simulink model "system_simulink-1"  (R2021b)
settings: Solver=ode45  StartTime=0.0  StopTime=20  RelTol=1e-3  EnableMultiTasking=on
undefined symbols (not defined in the file): dynamic_pre_comp, K, k_d, static_compensator
settings Model: Creator=Cabral  LastModifiedBy=Mohammad masih
settings SolverCC: AlgebraicLoopSolver=TrustRegion
settings DataIOCC: LimitDataPoints=on  SaveFormat=Array  SignalLoggingSaveFormat=ModelDataLogs  ReturnWorkspaceOutputs=off
settings OptimizationCC: ExpressionDepthLimit=2147483647  InitFltsAndDblsToZero=on  LifeSpan=inf
settings DebuggingCC: SaveWithParameterizedLinksMsg=none  UnderspecifiedInitializationDetection=Classic  MergeDetectMultiDrivingBlocksExec=none  SignalResolutionControl=TryResolveAllWithWarning  SolverPrmCheckMsg=warning  MultiTaskDSMMsg=warning  MultiTaskCondExecSysMsg=none  FcnCallInpInsideContextMsg=warning  StateNameClashWarn=warning  SFUnexpectedBacktrackingDiag=warning  SFNoUnconditionalDefaultTransitionDiag=warning  SFExecutionAtInitializationDiag=none  SFMachineParentedDataDiag=warning  ArithmeticOperatorsInVariantConditions=warning
settings HardwareCC: ProdBitPerPointer=32  ProdBitPerSizeT=32  ProdBitPerPtrDiffT=32  ProdLargestAtomicFloat=None  ProdIntDivRoundTo=Undefined  ProdEndianess=Unspecified  ProdWordSize=32  ProdHWDeviceType=32-bit Generic
settings ModelReferenceCC: PropagateSignalLabelsOutOfModel=off
settings SFSimCC: SimUseLocalCustomCode=off  SimParseCustomCode=off  CustomCodeUndefinedFunction=UseInterfaceOnly
settings RTWCC: RTWUseLocalCustomCode=off
settings CodeAppCC: StateflowObjectComments=on
settings GRTTargetCC: TargetFcnLib=ansi_tfl_tmw.mat  TargetLangStandard=C89/C90 (ANSI)  CombineOutputUpdateFcns=off  GRTInterface=on
settings ConfigComp: CovMetricSettings=dw  CovSaveCumulativeToWorkspaceVar=on  CovSaveSingleToWorkspaceVar=on  CovExternalEMLEnable=off

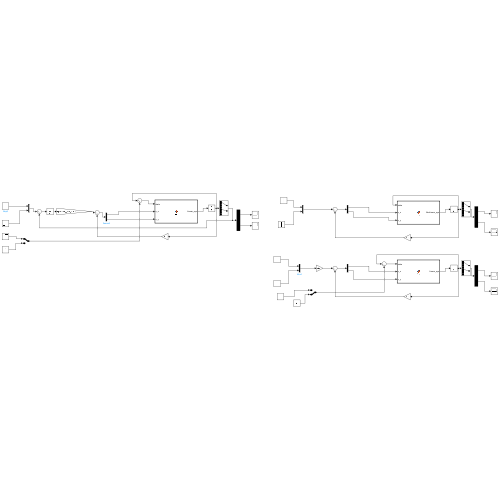
[thumbnail: Simulink's stored preview of the top-level diagram]
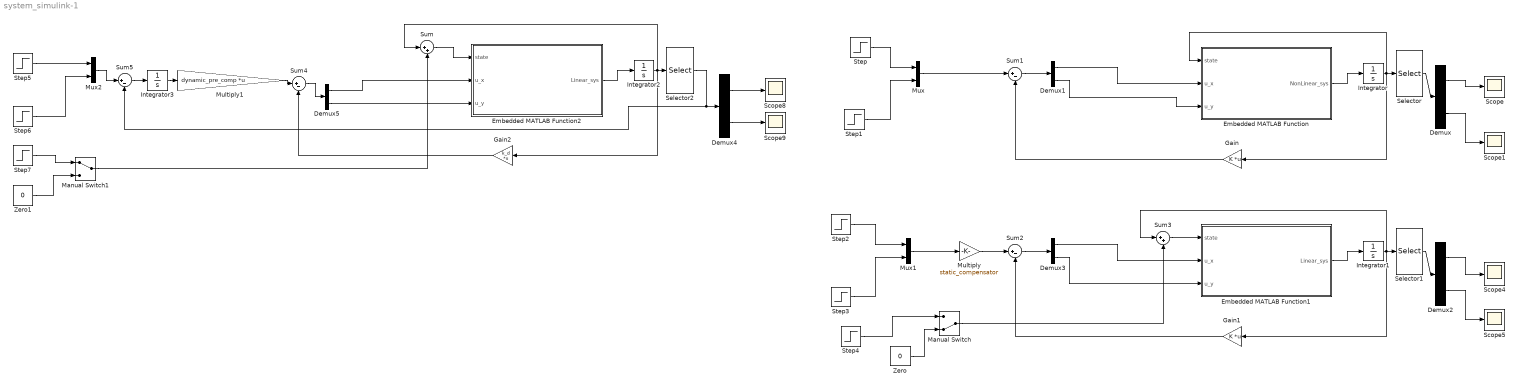
== system system_simulink-1 ==
  Demux{,1..5} (6 alike) : Demux  Outputs=[1 1]
  Embedded MATLAB Function : MATLAB Function  TreatAsAtomicUnit=on
  Embedded MATLAB Function1 : MATLAB Function  TreatAsAtomicUnit=on
  Embedded MATLAB Function2 : MATLAB Function  TreatAsAtomicUnit=on
  Gain : Gain  Gain=K  Multiplication=Matrix(K*u)
  Gain1 : Gain  Gain=K  Multiplication=Matrix(K*u)
  Gain2 : Gain  Gain=k_d  Multiplication=Matrix(K*u)
  Integrator : Integrator  InitialCondition=[0 0 0 0 0 0 0 0]
  Integrator1 : Integrator  InitialCondition=[0 0 0 0 0 0 0 0]
  Integrator2 : Integrator  InitialCondition=[0 0 0 0 0 0 0 0]
  Integrator3 : Integrator
  Manual Switch : ManualSwitch  CurrentSetting=0
  Manual Switch1 : ManualSwitch
  Multiply : Gain  Gain=static_compensator
  Multiply1 : Gain  Gain=dynamic_pre_comp  Multiplication=Matrix(K*u)
  Mux : Mux  Inputs=2
  Mux1 : Mux  Inputs=2
  Mux2 : Mux  Inputs=2
  Scope{,1,4..5,8..9} (6 alike) : Scope
  Selector : Selector  InputPortWidth=8  IndexOptions=Index vector (dialog)  Indices=[1 5]  OutputSizes=1
  Selector1 : Selector  InputPortWidth=8  IndexOptions=Index vector (dialog)  Indices=[1 5]  OutputSizes=1
  Selector2 : Selector  InputPortWidth=8  IndexOptions=Index vector (dialog)  Indices=[1 5]  OutputSizes=1
  Step{,1..3,5..7} (7 alike) : Step  SampleTime=0
  Step4 : Step  After=10  SampleTime=0
  Sum : Sum  Inputs=|++
  Sum{1..2,4..5} (4 alike) : Sum  Inputs=|+-
  Sum3 : Sum  Inputs=|++
  Zero : Constant  Value=0  OutDataTypeStr=Inherit: Inherit via back propagation
  Zero1 : Constant  Value=0  OutDataTypeStr=Inherit: Inherit via back propagation
  wires:
  Integrator/1 -> Gain/1, Selector/1, Embedded MATLAB Function/1(state)
  Selector/1 -> Demux/1
  Demux/2 -> Scope1/1
  Embedded MATLAB Function/1(NonLinear_sys) -> Integrator/1
  Demux/1 -> Scope/1
  Step/1 -> Mux/1
  Step1/1 -> Mux/2
  Sum1/1 -> Demux1/1
  Demux1/1 -> Embedded MATLAB Function/2(u_x)
  Demux1/2 -> Embedded MATLAB Function/3(u_y)
  Gain/1 -> Sum1/2
  Mux/1 -> Sum1/1
  Demux3/1 -> Embedded MATLAB Function1/2(u_x)
  Demux2/1 -> Scope4/1
  Sum2/1 -> Demux3/1
  Gain1/1 -> Sum2/2
  Step3/1 -> Mux1/2
  Demux3/2 -> Embedded MATLAB Function1/3(u_y)
  Integrator1/1 -> Sum3/1, Gain1/1, Selector1/1
  Demux2/2 -> Scope5/1
  Selector1/1 -> Demux2/1
  Embedded MATLAB Function1/1(Linear_sys) -> Integrator1/1
  Step2/1 -> Mux1/1
  Multiply/1 -> Sum2/1
  Step4/1 -> Manual Switch/1
  Zero/1 -> Manual Switch/2
  Zero1/1 -> Manual Switch1/2
  Step6/1 -> Mux2/2
  Demux4/2 -> Scope9/1
  Selector2/1 -> Demux4/1, Sum5/2
  Mux2/1 -> Sum5/1
  Sum4/1 -> Demux5/1
  Step7/1 -> Manual Switch1/1
  Demux5/2 -> Embedded MATLAB Function2/3(u_y)
  Step5/1 -> Mux2/1
  Demux5/1 -> Embedded MATLAB Function2/2(u_x)
  Gain2/1 -> Sum4/2
  Integrator2/1 -> Sum/1, Gain2/1, Selector2/1
  Demux4/1 -> Scope8/1
  Embedded MATLAB Function2/1(Linear_sys) -> Integrator2/1
  Sum5/1 -> Integrator3/1
  Integrator3/1 -> Multiply1/1
  Multiply1/1 -> Sum4/1
  Mux1/1 -> Multiply/1
  Sum/1 -> Embedded MATLAB Function2/1(state)
  Manual Switch1/1 -> Sum/2
  Sum3/1 -> Embedded MATLAB Function1/1(state)
  Manual Switch/1 -> Sum3/2

== matlab function system_simulink-1/Embedded MATLAB Function ==
  data: state input; u_x input; u_y input; NonLinear_sys output
function NonLinear_sys= fcn(state,u_x,u_y)
% constants
m = 0.11;
Ib = 1.76e-5;
rb = 0.02;

b = m/ (m + Ib/ rb^2)
g = 9.81;

x = state(1);
x_dot = state(2);
alfa = state(3);
alfa_dot = state(4);
y = state(5);
y_dot = state(6);
beta = state(7);
beta_dot = state(8);
if(alfa>1.57)
    alfa=1.57
    alfa_dot=0
end

if(beta>1.57)
    beta=1.57
    beta_dot=0
end
x_dot_dot = b*(x*alfa_dot*alfa_dot+alfa_dot*y*beta_dot-g*sin(alfa));
alpha_dot_dot = u_x;
y_dot_dot=b*(y*beta_dot*beta_dot+x*alfa_dot*beta_dot-g*sin(beta));
beta_dot_dot=u_y;

NonLinear_sys = [x_dot; x_dot_dot ;alfa_dot; alpha_dot_dot; y_dot ; y_dot_dot ; beta_dot ; beta_dot_dot];

== matlab function system_simulink-1/Embedded MATLAB Function1 ==
  data: state input; u_x input; u_y input; Linear_sys output
function Linear_sys= fcn(state,u_x,u_y)

A = [    0    1.0000         0         0         0         0         0         0;
         0         0   -7.0071         0         0         0         0         0;
         0         0         0    1.0000         0         0         0         0;
         0         0         0         0         0         0         0         0;
         0         0         0         0         0    1.0000         0         0;
         0         0         0         0         0         0   -7.0071         0;
         0         0         0         0         0         0         0    1.0000;
         0         0         0         0         0         0         0         0];
B=[  0     0;
     0     0;
     0     0;
     1     0;
     0     0;
     0     0;
     0     0;
     0     1];


Linear_sys = A*state+B*[u_x;u_y];

== matlab function system_simulink-1/Embedded MATLAB Function2 ==
  data: state input; u_x input; u_y input; Linear_sys output
function Linear_sys= fcn(state,u_x,u_y)

A = [    0    1.0000         0         0         0         0         0         0;
         0         0   -7.0071         0         0         0         0         0;
         0         0         0    1.0000         0         0         0         0;
         0         0         0         0         0         0         0         0;
         0         0         0         0         0    1.0000         0         0;
         0         0         0         0         0         0   -7.0071         0;
         0         0         0         0         0         0         0    1.0000;
         0         0         0         0         0         0         0         0];
B=[  0     0;
     0     0;
     0     0;
     1     0;
     0     0;
     0     0;
     0     0;
     0     1];


Linear_sys = A*state+B*[u_x;u_y];
